simulink model "Assignment_4_kalmanFilter"  (R2019b)
settings: Solver=VariableStepAuto  StartTime=0.0  StopTime=10.0  RelTol=1e-3
undefined symbols (not defined in the file): A, B, C, K, Q_diag, Ts, x0
libraries: simulink x1
settings Model: Creator=Vishrant  LastModifiedBy=Vishrant
settings SolverCC: AlgebraicLoopSolver=LineSearch
settings DebuggingCC: AlgebraicLoopMsg=none

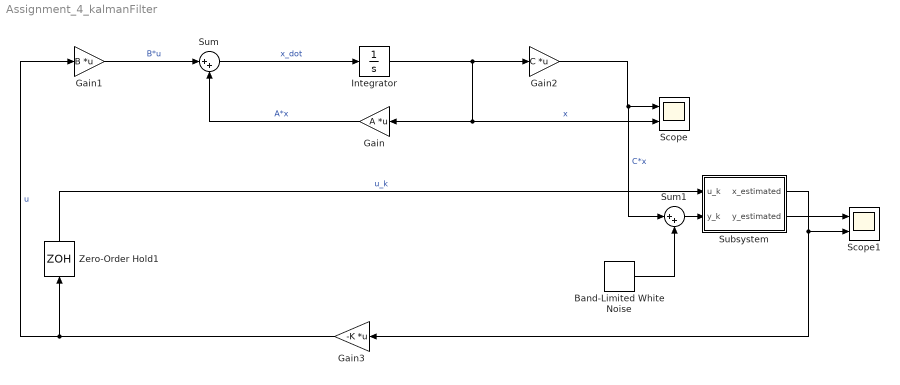
== system Assignment_4_kalmanFilter ==
  Band-Limited White Noise : simulink/Sources/Band-Limited White Noise  Cov=[0.005]  Ts=0.1  seed=[23341]
  Gain : Gain  Gain=A  Multiplication=Matrix(K*u)
  Gain1 : Gain  Gain=B  Multiplication=Matrix(K*u)
  Gain2 : Gain  Gain=C  Multiplication=Matrix(K*u)
  Gain3 : Gain  Gain=-K  Multiplication=Matrix(K*u)
  Integrator : Integrator  InitialCondition=x0
  Scope : Scope  NumInputPorts=2
  Scope1 : Scope  NumInputPorts=2
  Subsystem : Subsystem
  Sum : Sum  Inputs=|++
  Sum1 : Sum  Inputs=|++
  Zero-Order Hold1 : ZeroOrderHold  SampleTime=Ts
  wires:
  Gain2/1 -> Sum1/1, Scope/1  "C*x"
  Gain/1 -> Sum/2  "A*x"
  Integrator/1 -> Gain2/1, Gain/1, Scope/2  "x"
  Sum/1 -> Integrator/1  "x_dot"
  Gain1/1 -> Sum/1  "B*u"
  Gain3/1 -> Zero-Order Hold1/1, Gain1/1  "u"
  Zero-Order Hold1/1 -> Subsystem/1(u_k)  "u_k"
  Subsystem/1(x_estimated) -> Scope1/2, Gain3/1
  Sum1/1 -> Subsystem/2(y_k)
  Band-Limited White Noise/1 -> Sum1/2
  Subsystem/2(y_estimated) -> Scope1/1

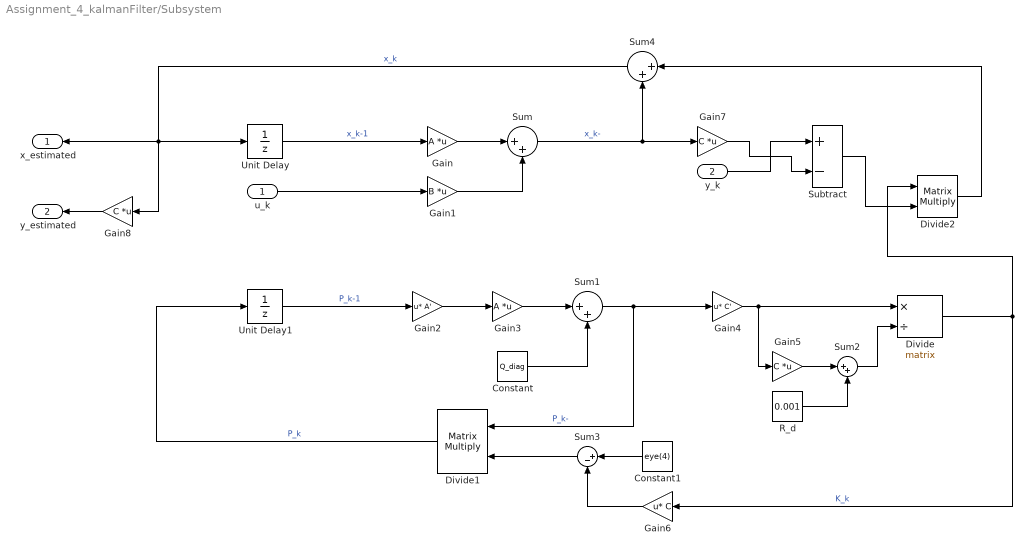
== system Assignment_4_kalmanFilter/Subsystem ==
  u_k : Inport
  y_k : Inport  Port=2
  Constant : Constant  Value=Q_diag
  Constant1 : Constant  Value=eye(4)
  Divide : Product  Inputs=*/  Multiplication=Matrix(*)
  Divide1 : Product  Multiplication=Matrix(*)
  Divide2 : Product  Multiplication=Matrix(*)
  Gain : Gain  Gain=A  Multiplication=Matrix(K*u)
  Gain1 : Gain  Gain=B  Multiplication=Matrix(K*u)
  Gain2 : Gain  Gain=A'  Multiplication=Matrix(u*K)
  Gain3 : Gain  Gain=A  Multiplication=Matrix(K*u)
  Gain4 : Gain  Gain=C'  Multiplication=Matrix(u*K)
  Gain5 : Gain  Gain=C  Multiplication=Matrix(K*u)
  Gain6 : Gain  Gain=C  Multiplication=Matrix(u*K)
  Gain7 : Gain  Gain=C  Multiplication=Matrix(K*u)
  Gain8 : Gain  Gain=C  Multiplication=Matrix(K*u)
  R_d : Constant  Value=0.001
  Subtract : Sum  Inputs=+-
  Sum{,1..2,4} (4 alike) : Sum  Inputs=|++
  Sum3 : Sum  Inputs=|+-
  Unit Delay : UnitDelay  SampleTime=-1  HasFrameUpgradeWarning=on
  Unit Delay1 : UnitDelay  SampleTime=-1  HasFrameUpgradeWarning=on
  x_estimated : Outport
  y_estimated : Outport  Port=2
  wires:
  u_k/1 -> Gain1/1
  Unit Delay/1 -> Gain/1  "x_k-1"
  Sum4/1 -> Gain8/1, x_estimated/1, Unit Delay/1  "x_k"
  Gain/1 -> Sum/1
  Gain1/1 -> Sum/2
  Sum/1 -> Gain7/1, Sum4/2  "x_k-"
  Unit Delay1/1 -> Gain2/1  "P_k-1"
  Divide1/1 -> Unit Delay1/1  "P_k"
  Gain2/1 -> Gain3/1
  Gain3/1 -> Sum1/1
  Constant/1 -> Sum1/2
  Sum1/1 -> Divide1/1, Gain4/1  "P_k-"
  Gain4/1 -> Gain5/1, Divide/1
  Gain5/1 -> Sum2/1
  R_d/1 -> Sum2/2
  Sum2/1 -> Divide/2
  Divide/1 -> Gain6/1, Divide2/1  "K_k"
  Constant1/1 -> Sum3/1
  Gain6/1 -> Sum3/2
  Sum3/1 -> Divide1/2
  Divide2/1 -> Sum4/1
  Gain8/1 -> y_estimated/1
  Subtract/1 -> Divide2/2
  y_k/1 -> Subtract/1
  Gain7/1 -> Subtract/2
